simulink model "tfExploDiscrete"  (R2017b)
settings: Solver=VariableStepDiscrete  StartTime=0.0  StopTime=10  MaxStep=1e-4  RelTol=1e-3
libraries: powerlib x1
settings Model: Creator=bikulborthakur  LastModifiedBy=bikulborthakur

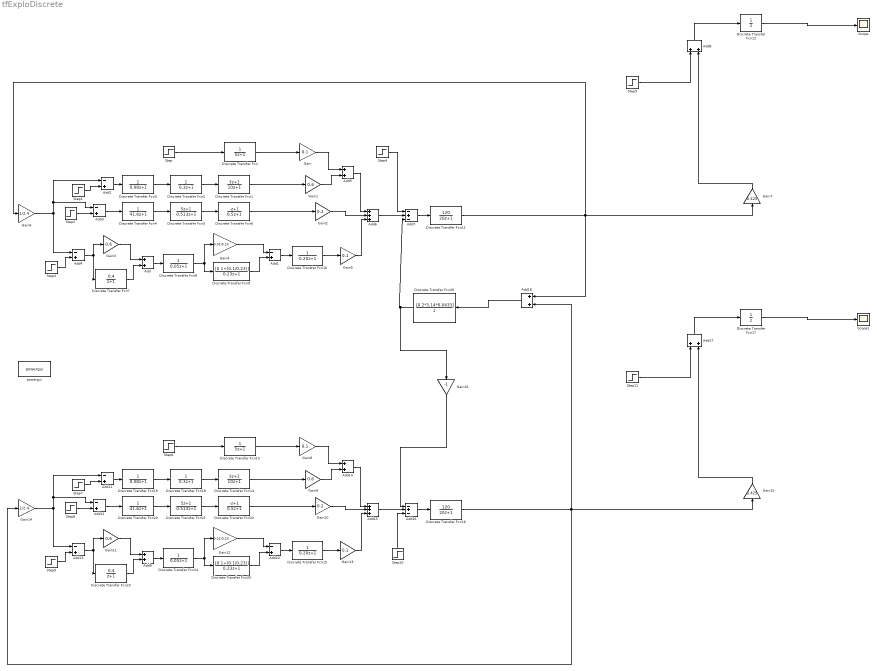
== system tfExploDiscrete ==
  Add{,5,8..9,14,17..18} (7 alike) : Sum
  Add{1..4,10..13} (8 alike) : Sum  Inputs=-+
  Add15 : Sum  Inputs=+++
  Add16 : Sum  Inputs=-+-
  Add6 : Sum  Inputs=+++
  Add7 : Sum  Inputs=-+-
  Discrete Transfer Fcn : DiscreteTransferFcn  Denominator=[5 1]  SampleTime=0.001
  Discrete Transfer Fcn1 : DiscreteTransferFcn  Numerator=[3 1]  Denominator=[10 1]  SampleTime=0.001
  Discrete Transfer Fcn10 : DiscreteTransferFcn  Numerator=[0 1]  Denominator=[0.20 1]  SampleTime=0.001
  Discrete Transfer Fcn11 : DiscreteTransferFcn  Numerator=[0 120]  Denominator=[20 1]  SampleTime=0.001
  Discrete Transfer Fcn12 : DiscreteTransferFcn  Numerator=[0 1]  Denominator=[1 0]  SampleTime=0.001
  Discrete Transfer Fcn13 : DiscreteTransferFcn  Denominator=[5 1]  SampleTime=0.001
  Discrete Transfer Fcn14 : DiscreteTransferFcn  Numerator=[3 1]  Denominator=[10 1]  SampleTime=0.001
  Discrete Transfer Fcn15 : DiscreteTransferFcn  Numerator=[0 1]  Denominator=[0.20 1]  SampleTime=0.001
  Discrete Transfer Fcn16 : DiscreteTransferFcn  Numerator=[0 120]  Denominator=[20 1]  SampleTime=0.001
  Discrete Transfer Fcn17 : DiscreteTransferFcn  Numerator=[0 1]  Denominator=[1 0]  SampleTime=0.001
  Discrete Transfer Fcn18 : DiscreteTransferFcn  Numerator=[0 1]  Denominator=[0.3 1]  SampleTime=0.001
  Discrete Transfer Fcn19 : DiscreteTransferFcn  Numerator=[0 1]  Denominator=[0.08 1]  SampleTime=0.001
  Discrete Transfer Fcn2 : DiscreteTransferFcn  Numerator=[0 1]  Denominator=[0.3 1]  SampleTime=0.001
  Discrete Transfer Fcn20 : DiscreteTransferFcn  Numerator=[0 1]  Denominator=[41.6 1]  SampleTime=0.001
  Discrete Transfer Fcn21 : DiscreteTransferFcn  Numerator=[5 1]  Denominator=[0.513 1]  SampleTime=0.001
  Discrete Transfer Fcn22 : DiscreteTransferFcn  Numerator=[-1 1]  Denominator=[0.5 1]  SampleTime=0.001
  Discrete Transfer Fcn23 : DiscreteTransferFcn  Numerator=[0 0.4]  Denominator=[1 1]  SampleTime=0.001
  Discrete Transfer Fcn24 : DiscreteTransferFcn  Numerator=[0 1]  Denominator=[0.05 1]  SampleTime=0.001
  Discrete Transfer Fcn25 : DiscreteTransferFcn  Numerator=[0 1+(0.1/0.23)]  Denominator=[ 0.23 1]
  Discrete Transfer Fcn26 : DiscreteTransferFcn  Numerator=[0 2*3.14*0.0433]  Denominator=[1 0]  SampleTime=0.001
  Discrete Transfer Fcn3 : DiscreteTransferFcn  Numerator=[0 1]  Denominator=[0.08 1]  SampleTime=0.001
  Discrete Transfer Fcn4 : DiscreteTransferFcn  Numerator=[0 1]  Denominator=[41.6 1]  SampleTime=0.001
  Discrete Transfer Fcn5 : DiscreteTransferFcn  Numerator=[5 1]  Denominator=[0.513 1]  SampleTime=0.001
  Discrete Transfer Fcn6 : DiscreteTransferFcn  Numerator=[-1 1]  Denominator=[0.5 1]  SampleTime=0.001
  Discrete Transfer Fcn7 : DiscreteTransferFcn  Numerator=[0 0.4]  Denominator=[1 1]  SampleTime=0.001
  Discrete Transfer Fcn8 : DiscreteTransferFcn  Numerator=[0 1]  Denominator=[0.05 1]  SampleTime=0.001
  Discrete Transfer Fcn9 : DiscreteTransferFcn  Numerator=[0 1+(0.1/0.23)]  Denominator=[ 0.23 1]
  Gain{,5,8,13} (4 alike) : Gain  Gain=0.1
  Gain{1,3,9,11} (4 alike) : Gain  Gain=0.6
  Gain10 : Gain  Gain=0.2
  Gain12 : Gain  Gain=0.01/0.23
  Gain14 : Gain  Gain=1/2.4
  Gain15 : Gain  Gain=0.425
  Gain16 : Gain  Gain=-1
  Gain2 : Gain  Gain=0.2
  Gain4 : Gain  Gain=0.01/0.23
  Gain6 : Gain  Gain=1/2.4
  Gain7 : Gain  Gain=0.425
  Scope : Scope
  Scope1 : Scope
  Step{,1..11} (12 alike) : Step  SampleTime=0
  powergui : powerlib/powergui  Priority=1  SimulationMode=Discrete  SampleTime=0.001  frequency=60  Iterations=50  frequencyindice=60  Pbase=100e6  ErrMax=1e-4  UnitsV=kV  UnitsW=MW  buscounter=0  FunctionMessages=off  echomessages=off  EnableUseOfTLC=off  CurrentSourceSwitches=off  DisableSnubberDevices=off  DisableRonSwitches=off  DisableVfSwitches=off  DisplayEquations=off  SolverType=Tustin/Backward Euler (TBE)  Interpol=off  ExternalGateDelay=off  methode=off  Ts=100  x0status=blocks  SPID=on  SwTol=0  HookPort=off  RestoreLinks=warning  ResistiveCurrentMeasurement=off  Frange=[0:2:500]  Ylog=off  Xlog=on  ShowGrid=off  save=off  variable=ZData  structure=0  ZoomFFT=off  StartTime=0.0  cycles=1  DisplayStyle=1  fundamental=60  FreqAxis=off  MaxFrequency=1000  frequencyindicesteady=1  RmsSteady=1  display=off
  wires:
  Discrete Transfer Fcn3/1 -> Discrete Transfer Fcn2/1
  Discrete Transfer Fcn2/1 -> Discrete Transfer Fcn1/1
  Discrete Transfer Fcn/1 -> Gain/1
  Step/1 -> Discrete Transfer Fcn/1
  Discrete Transfer Fcn4/1 -> Discrete Transfer Fcn5/1
  Discrete Transfer Fcn5/1 -> Discrete Transfer Fcn6/1
  Discrete Transfer Fcn1/1 -> Gain1/1
  Discrete Transfer Fcn6/1 -> Gain2/1
  Gain3/1 -> Add/1
  Discrete Transfer Fcn7/1 -> Add/2
  Add/1 -> Discrete Transfer Fcn8/1
  Discrete Transfer Fcn8/1 -> Discrete Transfer Fcn9/1, Gain4/1
  Gain4/1 -> Add1/1
  Discrete Transfer Fcn9/1 -> Add1/2
  Add2/1 -> Discrete Transfer Fcn3/1
  Add3/1 -> Discrete Transfer Fcn4/1
  Add4/1 -> Discrete Transfer Fcn7/1, Gain3/1
  Step1/1 -> Add2/2
  Step2/1 -> Add3/2
  Step3/1 -> Add4/2
  Gain6/1 -> Add4/1, Add3/1, Add2/1
  Add1/1 -> Discrete Transfer Fcn10/1
  Discrete Transfer Fcn10/1 -> Gain5/1
  Gain/1 -> Add5/1
  Gain1/1 -> Add5/2
  Add5/1 -> Add6/1
  Gain2/1 -> Add6/2
  Gain5/1 -> Add6/3
  Step4/1 -> Add7/1
  Add6/1 -> Add7/2
  Add7/1 -> Discrete Transfer Fcn11/1
  Discrete Transfer Fcn11/1 -> Add18/1, Gain6/1, Gain7/1
  Step5/1 -> Add8/1
  Gain7/1 -> Add8/2
  Add8/1 -> Discrete Transfer Fcn12/1
  Discrete Transfer Fcn12/1 -> Scope/1
  Add9/1 -> Discrete Transfer Fcn24/1
  Gain9/1 -> Add14/2
  Discrete Transfer Fcn22/1 -> Gain10/1
  Discrete Transfer Fcn13/1 -> Gain8/1
  Gain14/1 -> Add13/1, Add12/1, Add11/1
  Add17/1 -> Discrete Transfer Fcn17/1
  Add13/1 -> Discrete Transfer Fcn23/1, Gain11/1
  Discrete Transfer Fcn16/1 -> Add18/2, Gain14/1, Gain15/1
  Add15/1 -> Add16/2
  Discrete Transfer Fcn14/1 -> Gain9/1
  Gain13/1 -> Add15/3
  Gain11/1 -> Add9/1
  Step7/1 -> Add11/2
  Discrete Transfer Fcn18/1 -> Discrete Transfer Fcn14/1
  Discrete Transfer Fcn20/1 -> Discrete Transfer Fcn21/1
  Discrete Transfer Fcn23/1 -> Add9/2
  Discrete Transfer Fcn21/1 -> Discrete Transfer Fcn22/1
  Step6/1 -> Discrete Transfer Fcn13/1
  Discrete Transfer Fcn19/1 -> Discrete Transfer Fcn18/1
  Gain8/1 -> Add14/1
  Add16/1 -> Discrete Transfer Fcn16/1
  Gain12/1 -> Add10/1
  Discrete Transfer Fcn25/1 -> Add10/2
  Add14/1 -> Add15/1
  Step9/1 -> Add13/2
  Gain15/1 -> Add17/2
  Step11/1 -> Add17/1
  Discrete Transfer Fcn17/1 -> Scope1/1
  Step8/1 -> Add12/2
  Add12/1 -> Discrete Transfer Fcn20/1
  Gain10/1 -> Add15/2
  Add11/1 -> Discrete Transfer Fcn19/1
  Add10/1 -> Discrete Transfer Fcn15/1
  Discrete Transfer Fcn15/1 -> Gain13/1
  Discrete Transfer Fcn24/1 -> Discrete Transfer Fcn25/1, Gain12/1
  Add18/1 -> Discrete Transfer Fcn26/1
  Discrete Transfer Fcn26/1 -> Gain16/1, Add7/3
  Step10/1 -> Add16/3
  Gain16/1 -> Add16/1
